simulink model "BEML_EMU"  (R2019b)
settings: configuration reference "ConfigSet_SimIntegration" (kept outside this file)
model workspace (MAT data in the model file):
  BrakesSampleTime = 0.01
  ConfigSampleTime = 0.05
  CouplingSampleTime = 0.05
  DoorsSampleTime = 0.05
  DynamicsSampleTime = 0.001
  ElectricalSampleTime = 0.05
  PRM_SimIntegration : Simulink.Parameter (value not decoded)
  PantographSampleTime = 0.05
  PneumaticsSampleTime = 0.01
  SampleTime = 0.001
  TractionSampleTime = 0.01
undefined symbols (not defined in the file): Acceleration, AngularAcceleration, AngularVelocity, BrakeFadeEnable, Brakes, BrakeShoeCoefficientCalculationMethod, BrakeShoeFrictionCoeff, BrakeTemperatureEnable, Common, DampingAdjustmentDesignMass, DavisCoeffA1, DavisCoeffA2, DavisCoeffB1, DavisCoeffB2, DavisCoefficients, DavisCoeffLeadCarC, DavisCoeffTailCarC, DiscIntNeverNeededParam, Doors, DragCalculationMethod, Dynamics, Effects, Electrical, EnableDampingAdjustmentByMass, Environment, Equipment, ExternalEffects, H, HasMotor, HasPanto, HornActivation, IsFirstVehicle, IsLastVehicle, isLeft, IsNonCab, LateralJolt, Location, LongitudinalJolt, MaxVehicles, MotionBaseSafetyCutout, OrientationDCM, P, Pantograph, Pneumatics, PneumaticsPoweredPanto, R, Traction, Transform, Tuning, UnitConfig, Velocity, VerticalJolt, VerticalJoltDown, VigilanceIntervention
libraries: simulink x35, IOStateMachinesLib x26, TestBenchLib x6, LatchesLib x3, BEML_EMU_BrakesInput_Lib x1, BEML_EMU_CBTCInterface_Lib x1, BEML_EMU_Couplers_Lib x1, BEML_EMU_DoorsInput_Lib x1, BEML_EMU_DynamicsInput_Lib x1, BEML_EMU_ElectricalInput_Lib x1, BEML_EMU_PantographInput_Lib x1, BEML_EMU_PneumaticsInput_Lib x1
(part 3 of 6)

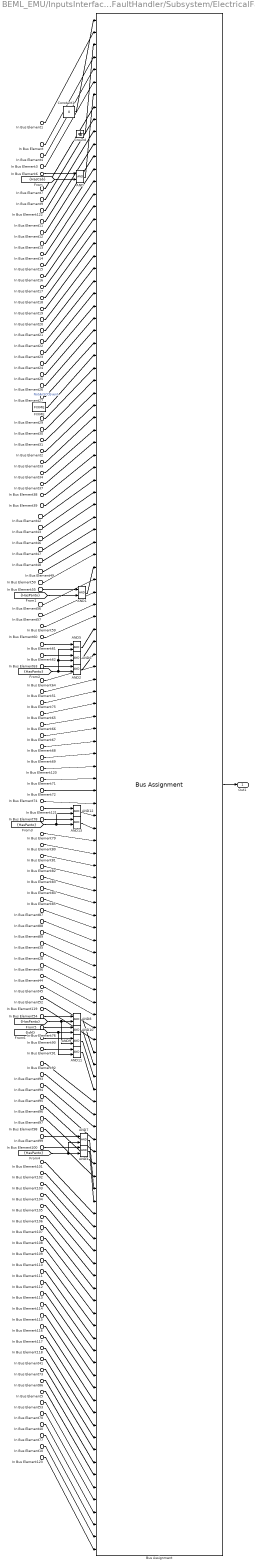
== system BEML_EMU/InputsInterface/FaultHandler/Subsystem/ElectricalFaults ==
  In Bus Element4 : Inport  PortName=TrainFaults  Element=FWDREVTrainLineMismatch
  In Bus Element6 : Inport  PortName=TrainFaults  Element=LowMRPressure
  In Bus Element7 : Inport  PortName=TrainFaults  Element=ReverseMotionInForwardCommand
  In Bus Element9 : Inport  PortName=TrainFaults  Element=InternalFireAlarmTLActive
  In Bus Element11 : Inport  PortName=TrainFaults  Element=TractionCutModeSelectorInATPATOUTO
  In Bus Element12 : Inport  PortName=TrainFaults  Element=DamagedOHE
  In Bus Element13 : Inport  PortName=TrainFaults  Element=DoorsNotOpeningFromDOPBOP1
  In Bus Element14 : Inport  PortName=TrainFaults  Element=DepotSignalMalfunction
  In Bus Element15 : Inport  PortName=TrainFaults  Element=TrackCircuitOccupied
  In Bus Element16 : Inport  PortName=TrainFaults  Element=MainSignalSwitchesToRed
  In Bus Element17 : Inport  PortName=TrainFaults  Element=PlatformScreenDoorNotWorking
  In Bus Element18 : Inport  PortName=TrainFaults  Element=TrainGettingZeroSpeedOrder
  In Bus Element19 : Inport  PortName=TrainFaults  Element=ATCEBUnableToReset
  In Bus Element20 : Inport  PortName=TrainFaults  Element=TrainOvershootATCNotAllowingReverseAlignment
  In Bus Element21 : Inport  PortName=TrainFaults  Element=FSBAppliedAt10KMPH
  In Bus Element122 : Inport  PortName=TrainFaults  Element=FDUFaultAlarmTLActive
  In Bus Element1 : Inport  Port=2  PortName=VehicleFaults  Element=PantographDownForADDIntervention
  In Bus Element : Inport  Port=2  PortName=VehicleFaults  Element=PantographRaiseFailure
  In Bus Element3 : Inport  Port=2  PortName=VehicleFaults  Element=CCDetectDetrainmentDoorOpen
  In Bus Element22 : Inport  Port=2  PortName=VehicleFaults  Element=HVAC1SupplyFanMPCBTrip
  In Bus Element23 : Inport  Port=2  PortName=VehicleFaults  Element=HVAC1EmergencyInverterTrip
  In Bus Element24 : Inport  Port=2  PortName=VehicleFaults  Element=HVAC1RCCBTrip
  In Bus Element25 : Inport  Port=2  PortName=VehicleFaults  Element=HVAC1FireMode
  In Bus Element26 : Inport  Port=2  PortName=VehicleFaults  Element=HVAC1ExternalSmokeMode
  In Bus Element27 : Inport  Port=2  PortName=VehicleFaults  Element=HVAC1ReducedMode
  In Bus Element29 : Inport  Port=2  PortName=VehicleFaults  Element=WFLFailure
  In Bus Element30 : Inport  Port=2  PortName=VehicleFaults  Element=ODDFailure
  In Bus Element31 : Inport  Port=2  PortName=VehicleFaults  Element=ObstacleDetectedRightSide
  In Bus Element33 : Inport  Port=2  PortName=VehicleFaults  Element=CouplingCircuitNotPowered
  In Bus Element34 : Inport  Port=2  PortName=VehicleFaults  Element=CabEnablingCircuitBreakerTripped
  In Bus Element37 : Inport  Port=2  PortName=VehicleFaults  Element=OHLHighVoltageLevel3
  In Bus Element38 : Inport  Port=2  PortName=VehicleFaults  Element=OHLLowVoltageLevel2
  In Bus Element39 : Inport  Port=2  PortName=VehicleFaults  Element=LineConverterOverCurrentLevel2
  In Bus Element42 : Inport  Port=2  PortName=VehicleFaults  Element=LineConverterIGBTFailure
  In Bus Element43 : Inport  Port=2  PortName=VehicleFaults  Element=DC110VLowVoltage
  In Bus Element46 : Inport  Port=2  PortName=VehicleFaults  Element=OverTemperatureOfInverterPowerUnit
  In Bus Element47 : Inport  Port=2  PortName=VehicleFaults  Element=OverTemperatureOfConverterPowerUnit
  In Bus Element48 : Inport  Port=2  PortName=VehicleFaults  Element=AKOpenFailure
  In Bus Element49 : Inport  Port=2  PortName=VehicleFaults  Element=KOpenFailure
  In Bus Element50 : Inport  Port=2  PortName=VehicleFaults  Element=MainCircuitEarthFaultLevel2
  In Bus Element55 : Inport  Port=2  PortName=VehicleFaults  Element=VCBOpenedByCI
  In Bus Element56 : Inport  Port=2  PortName=VehicleFaults  Element=PantographDownForBUVDRIntervention
  In Bus Element57 : Inport  Port=2  PortName=VehicleFaults  Element=PantographCircuitNotEnergized
  In Bus Element59 : Inport  Port=2  PortName=VehicleFaults  Element=TransformerOilPressureTooLow
  In Bus Element60 : Inport  Port=2  PortName=VehicleFaults  Element=TransformerOilTemperatureTooHigh
  In Bus Element61 : Inport  Port=2  PortName=VehicleFaults  Element=VCBOpenedByACOvercurrent
  In Bus Element62 : Inport  Port=2  PortName=VehicleFaults  Element=VCBOpenedByMTrProtection
  In Bus Element63 : Inport  Port=2  PortName=VehicleFaults  Element=VCBOpenedByAPS
  In Bus Element64 : Inport  Port=2  PortName=VehicleFaults  Element=PantographLoweringFailure
  In Bus Element65 : Inport  Port=2  PortName=VehicleFaults  Element=MCB110VDCGroupTripped
  In Bus Element66 : Inport  Port=2  PortName=VehicleFaults  Element=MechanicalCouplerRelayFault
  In Bus Element67 : Inport  Port=2  PortName=VehicleFaults  Element=BatteryFuseBlown
  In Bus Element68 : Inport  Port=2  PortName=VehicleFaults  Element=BICContactorActivationFault
  In Bus Element69 : Inport  Port=2  PortName=VehicleFaults  Element=LowBatteryVoltageAlarm
  In Bus Element71 : Inport  Port=2  PortName=VehicleFaults  Element=MCBHVACGroupTripped
  In Bus Element72 : Inport  Port=2  PortName=VehicleFaults  Element=HVAC1MajorFault
  In Bus Element74 : Inport  Port=2  PortName=VehicleFaults  Element=MCBSignalingGroupTripped
  In Bus Element78 : Inport  Port=2  PortName=VehicleFaults  Element=APSCircuitBreakerTripped
  In Bus Element79 : Inport  Port=2  PortName=VehicleFaults  Element=SmokeAlarmCABArea
  In Bus Element80 : Inport  Port=2  PortName=VehicleFaults  Element=HeatAlarmEDB
  In Bus Element81 : Inport  Port=2  PortName=VehicleFaults  Element=TrainRadioFailure
  In Bus Element82 : Inport  Port=2  PortName=VehicleFaults  Element=PEA1AlarmActive
  In Bus Element83 : Inport  Port=2  PortName=VehicleFaults  Element=PEA1CallNotAcknowledged
  In Bus Element84 : Inport  Port=2  PortName=VehicleFaults  Element=PEA1Failure
  In Bus Element85 : Inport  Port=2  PortName=VehicleFaults  Element=MCBPAGroupOpen
  In Bus Element87 : Inport  Port=2  PortName=VehicleFaults  Element=CommunicationErrorRIO1RIO2
  In Bus Element88 : Inport  Port=2  PortName=VehicleFaults  Element=MCBTCMSGroupTripped
  In Bus Element89 : Inport  Port=2  PortName=VehicleFaults  Element=ER1MajorFault
  In Bus Element51 : Inport  Port=2  PortName=VehicleFaults  Element=MCBBrakeGroupTripped
  In Bus Element75 : Inport  Port=2  PortName=VehicleFaults  Element=MCBDoorGroupTripped
  In Bus Element35 : Inport  Port=2  PortName=VehicleFaults  Element=EDNORDeactivatedInRunningTrain
  In Bus Element28 : Inport  Port=2  PortName=VehicleFaults  Element=AllDoorCloseIndicatorNotWorking
  In Bus Element36 : Inport  Port=2  PortName=VehicleFaults  Element=TrainDoorLockedClosedRelayFailure
  In Bus Element44 : Inport  Port=2  PortName=VehicleFaults  Element=WipersNotWorking
  In Bus Element45 : Inport  Port=2  PortName=VehicleFaults  Element=FloodLightNotWorking
  In Bus Element52 : Inport  Port=2  PortName=VehicleFaults  Element=ShutdownFailureVCBOpening
  In Bus Element54 : Inport  Port=2  PortName=VehicleFaults  Element=ExteriorLight1CBTripped
  In Bus Element76 : Inport  Port=2  PortName=VehicleFaults  Element=ExteriorLight2CBTripped
  In Bus Element90 : Inport  Port=2  PortName=VehicleFaults  Element=InteriorLight1CBTripped
  In Bus Element91 : Inport  Port=2  PortName=VehicleFaults  Element=InteriorLight2CBTripped
  In Bus Element92 : Inport  Port=2  PortName=VehicleFaults  Element=CMCContactorActivationFailure
  In Bus Element93 : Inport  Port=2  PortName=VehicleFaults  Element=CMCContactorDeactivationFailure
  In Bus Element94 : Inport  Port=2  PortName=VehicleFaults  Element=APSGroup1Failure
  In Bus Element95 : Inport  Port=2  PortName=VehicleFaults  Element=APSGroup1Isolated
  In Bus Element96 : Inport  Port=2  PortName=VehicleFaults  Element=BCGGroup1Failure
  In Bus Element97 : Inport  Port=2  PortName=VehicleFaults  Element=BCGGroup1IsolationFailure
  In Bus Element98 : Inport  Port=2  PortName=VehicleFaults  Element=BCGGroup1Isolated
  In Bus Element99 : Inport  Port=2  PortName=VehicleFaults  Element=VCBMissingClosing
  In Bus Element100 : Inport  Port=2  PortName=VehicleFaults  Element=VCBMissingOpening
  In Bus Element101 : Inport  Port=2  PortName=VehicleFaults  Element=HeadlightFailure
  In Bus Element102 : Inport  Port=2  PortName=VehicleFaults  Element=HornBlowsContinuously
  In Bus Element103 : Inport  Port=2  PortName=VehicleFaults  Element=LineVoltageIndicatorNotWorking
  In Bus Element104 : Inport  Port=2  PortName=VehicleFaults  Element=OtherCabOccupiedIndicatorFaulty
  In Bus Element105 : Inport  Port=2  PortName=VehicleFaults  Element=DoorClosePBOP1NotWorking
  In Bus Element106 : Inport  Port=2  PortName=VehicleFaults  Element=EmergencyBrakePBOP1NotWorking
  In Bus Element107 : Inport  Port=2  PortName=VehicleFaults  Element=DoorCloseAnnouncementPBNotWorking
  In Bus Element108 : Inport  Port=2  PortName=VehicleFaults  Element=FailureOfTrainborneATCEquipment
  In Bus Element109 : Inport  Port=2  PortName=VehicleFaults  Element=DMIFailure
  In Bus Element110 : Inport  Port=2  PortName=VehicleFaults  Element=TransformerOilLevelLow
  In Bus Element111 : Inport  Port=2  PortName=VehicleFaults  Element=TransformerOilFlowWarning
  In Bus Element112 : Inport  Port=2  PortName=VehicleFaults  Element=TransformerOilPressureWarning
  In Bus Element113 : Inport  Port=2  PortName=VehicleFaults  Element=TransformerOilTemperatureHigh
  In Bus Element114 : Inport  Port=2  PortName=VehicleFaults  Element=PCUFailure
  In Bus Element115 : Inport  Port=2  PortName=VehicleFaults  Element=PEA2Failure
  In Bus Element116 : Inport  Port=2  PortName=VehicleFaults  Element=PEA3Failure
  In Bus Element117 : Inport  Port=2  PortName=VehicleFaults  Element=SCU2Failure
  In Bus Element118 : Inport  Port=2  PortName=VehicleFaults  Element=EBNotReleased
  In Bus Element41 : Inport  Port=2  PortName=VehicleFaults  Element=CIMicroprocessorAbnormal
  In Bus Element73 : Inport  Port=2  PortName=VehicleFaults  Element=CILocalCommunicationFailure
  In Bus Element86 : Inport  Port=2  PortName=VehicleFaults  Element=TransformerOilLevelTooLow
  In Bus Element119 : Inport  Port=2  PortName=VehicleFaults  Element=MCBLightGroupSaloonTripped
  In Bus Element120 : Inport  Port=2  PortName=VehicleFaults  Element=MCBLightGroupTripped
  In Bus Element121 : Inport  Port=2  PortName=VehicleFaults  Element=MCBAPSGroupTripped
  In Bus Element5 : Inport  Port=2  PortName=VehicleFaults  Element=PantographRisingMissing
  In Bus Element53 : Inport  Port=2  PortName=VehicleFaults  Element=PantographLoweringMissing
  In Bus Element70 : Inport  Port=2  PortName=VehicleFaults  Element=PantographRisingInhibited
  In Bus Element40 : Inport  Port=2  PortName=VehicleFaults  Element=CIFailure
  In Bus Element77 : Inport  Port=2  PortName=VehicleFaults  Element=CIIsolated
  In Bus Element10 : Inport  Port=2  PortName=VehicleFaults  Element=EmergencyBrakeDueToEBPB
  In Bus Element123 : Inport  Port=2  PortName=VehicleFaults  Element=EmergencyBrakeDueDeadman
  In Bus Element2 : Inport  Port=2  PortName=VehicleFaults  Element=DerailmentDetectedRightSide
  AND{,1..2,4..13} (13 alike) : Logic  AllPortsSameDT=off  OutDataTypeStr=boolean
  Bus Assignment : BusAssignment  AssignedSignals=PantographDownForADDIntervention,PantographDownForORDIntervention,PantographRisingFailure,FwdRevTrainLineMismatch,CCDetectedEmerDoorOpen,LowMRPressure,ReverseMotionInForwardCommand,InternalFireAlarmTLActive,FDUFailure,TractionCutModeSelectorInATPATOUTO,DamagedOHE,DoorsNotOpeningFromDOPBOP1,DepotSignalMalfunction,TrackCircuitOccupied,MainSignalSwitchesToRed,PlatformScreenDoorNotWorking,TrainGettingZeroSpeedOrder,ATCEBUnableToReset,TrainOvershootATCNotAllowingReverseAlignment,FSBAppliedAt10KMPH,HVAC1SupplyFanMPCBTrip,HVAC1EmergencyInverterTrip,HVAC1RCCBTrip,HVAC1FireMode,HVAC1ExternalSmokeMode,HVAC1ReducedMode,CabSaloonPartitionDoorOpen,WFLFailure,ODDFailure,ObstacleDetectedRightSide,DerailmentDetectedRightSide,CouplingCircuitNotPowered,CabEnablingCircuitBreakerTripped,OHLHighVoltageLevel3,OHLLowVoltageLevel2,LineConverterOverCurrentLevel2,LineConverterIGBTFailure,DC110VLowVoltage,OverTemperatureOfInverterPowerUnit,OverTemperatureOfConverterPowerUnit,AKOpenFailure,KOpenFailure,MainCircuitEarthFaultLevel2,VCBOpenedByCI,PantographDownForBUVDRIntervention,PantographCircuitNotEnergized,TransformerOilPressureTooLow,TransformerOilTemperatureTooHigh,VCBOpenedByACOvercurrent,VCBOpenedByMTrProtection,VCBOpenedByAPS,PantographLoweringFailure,MCBBrakeGroupTripped,MCBDoorGroupTripped,MCB110VDCGroupTripped,MechanicalCouplerRelayFault,BatteryFuseBlown,BICContactorActivationFault,LowBatteryVoltageAlarm,LightGroupMCBTripped,MCBHVACGroupTripped,HVAC1MajorFault,MCBSignalingGroupTripped,APSMCBGroupTripped,APSCircuitBreakerTripped,SmokeAlarmCABArea,HeatAlarmEDB,TrainRadioFailure,PEA1AlarmActive,PEA1CallNotAcknowledged,PEA1Failure,MCBPAGroupOpen,CommunicationErrorRIO1RIO2,MCBTCMSGroupTripped,ER1MajorFault,EmerDoorNotOpenRelayDeactivated,AllDoorCloseIndicatorNotWorking,TrainDoorLockedClosedRelayFailure,WipersNotWorking,FloodLightNotWorking,ShutdownFailureVCBOpening,LightGroupSaloonMCBTripped,ExteriorLight1CBTripped,ExteriorLight2CBTripped,InteriorLight1CBTripped,InteriorLight2CBTripped,CMCContactorActivationFailure,CMCContactorDeactivationFailure,APSGroup1Failure,APSGroup1Isolated,BCGGroup1Failure,BCGGroup1IsolationFailure,BCGGroup1Isolated,VCBMissingClosing,VCBMissingOpening,HeadlightFailure,HornBlowsContinuously,LineVoltageIndicatorNotWorking,OtherCabOccupiedIndicatorFaulty,DoorClosePBOP1NotWorking,EmergencyBrakePBOP1NotWorking,DoorCloseAnnouncementPBNotWorking,ATCFailure,DMIFailure,TransformerOilLevelLow,TransformerOilFlowWarning,TransformerOilPressureWarning,TransformerOilTemperatureHigh,PCUFailure,PEA2Failure,PEA3Failure,SCU2Failure,EBNotReleased,CIMicroprocessorAbnormal,CILocalCommunicationFailure,TransformerOilLevelTooLow,PantographRisingMissing,PantographLoweringMissing,PantographRisingInhibited,CIFailure,CIIsolated,EmergencyBrakeDueToEBPB,EmergencyBrakeDueDeadman
  Constant1 : Constant  Value=0  OutDataTypeStr=Bus: BD_ElectricalSystem_In_Faults
  FIXME : TestBenchLib/FIXME
      settings: SourceProductName=Sydac Utilities
  Ground : Ground
  Out1 : Outport
  wires:
  Bus Assignment/1 -> Out1/1
  Constant1/1 -> Bus Assignment/1
  In Bus Element1/1 -> Bus Assignment/2
  In Bus Element/1 -> Bus Assignment/4
  In Bus Element3/1 -> Bus Assignment/6
  In Bus Element6/1 -> AND/1
  AND/1 -> Bus Assignment/7
  [HasCab] -> AND/2
  In Bus Element55/1 -> AND1/1
  [HasPanto] -> AND1/2
  In Bus Element7/1 -> Bus Assignment/8
  In Bus Element61/1 -> AND5/1
  In Bus Element78/1 -> AND13/1
  In Bus Element99/1 -> AND7/1
  In Bus Element62/1 -> AND6/1
  [HasPanto] -> AND9/2, AND8/2
  In Bus Element54/1 -> AND8/1
  [HasPanto] -> AND12/2, AND13/2
  [HasPanto] -> AND6/2, AND5/2, AND2/2
  [HasPanto] -> AND7/2, AND4/2
  [IsM] -> AND11/2, AND10/2
  In Bus Element91/1 -> AND11/1
  In Bus Element121/1 -> AND12/1
  In Bus Element76/1 -> AND10/1
  In Bus Element90/1 -> AND9/1
  In Bus Element63/1 -> AND2/1
  In Bus Element100/1 -> AND4/1
  In Bus Element2/1 -> Bus Assignment/32
  FIXME/1 -> Bus Assignment/28  "NotAnSCCEvent"
  In Bus Element9/1 -> Bus Assignment/9
  In Bus Element122/1 -> Bus Assignment/10
  In Bus Element11/1 -> Bus Assignment/11
  In Bus Element12/1 -> Bus Assignment/12
  In Bus Element13/1 -> Bus Assignment/13
  In Bus Element14/1 -> Bus Assignment/14
  In Bus Element15/1 -> Bus Assignment/15
  In Bus Element16/1 -> Bus Assignment/16
  In Bus Element17/1 -> Bus Assignment/17
  In Bus Element18/1 -> Bus Assignment/18
  In Bus Element19/1 -> Bus Assignment/19
  In Bus Element20/1 -> Bus Assignment/20
  In Bus Element21/1 -> Bus Assignment/21
  In Bus Element22/1 -> Bus Assignment/22
  In Bus Element23/1 -> Bus Assignment/23
  In Bus Element24/1 -> Bus Assignment/24
  In Bus Element25/1 -> Bus Assignment/25
  In Bus Element26/1 -> Bus Assignment/26
  In Bus Element27/1 -> Bus Assignment/27
  In Bus Element29/1 -> Bus Assignment/29
  In Bus Element30/1 -> Bus Assignment/30
  In Bus Element33/1 -> Bus Assignment/33
  In Bus Element34/1 -> Bus Assignment/34
  In Bus Element37/1 -> Bus Assignment/35
  In Bus Element38/1 -> Bus Assignment/36
  In Bus Element39/1 -> Bus Assignment/37
  In Bus Element42/1 -> Bus Assignment/38
  In Bus Element43/1 -> Bus Assignment/39
  In Bus Element46/1 -> Bus Assignment/40
  In Bus Element47/1 -> Bus Assignment/41
  In Bus Element48/1 -> Bus Assignment/42
  In Bus Element49/1 -> Bus Assignment/43
  In Bus Element50/1 -> Bus Assignment/44
  AND1/1 -> Bus Assignment/45
  AND5/1 -> Bus Assignment/50
  AND6/1 -> Bus Assignment/51
  AND2/1 -> Bus Assignment/52
  In Bus Element59/1 -> Bus Assignment/48
  In Bus Element60/1 -> Bus Assignment/49
  In Bus Element56/1 -> Bus Assignment/46
  In Bus Element57/1 -> Bus Assignment/47
  In Bus Element64/1 -> Bus Assignment/53
  In Bus Element51/1 -> Bus Assignment/54
  In Bus Element75/1 -> Bus Assignment/55
  In Bus Element65/1 -> Bus Assignment/56
  In Bus Element66/1 -> Bus Assignment/57
  In Bus Element67/1 -> Bus Assignment/58
  In Bus Element68/1 -> Bus Assignment/59
  In Bus Element69/1 -> Bus Assignment/60
  In Bus Element120/1 -> Bus Assignment/61
  In Bus Element71/1 -> Bus Assignment/62
  In Bus Element72/1 -> Bus Assignment/63
  In Bus Element74/1 -> Bus Assignment/64
  AND12/1 -> Bus Assignment/65
  AND13/1 -> Bus Assignment/66
  AND8/1 -> Bus Assignment/84
  AND10/1 -> Bus Assignment/85
  AND9/1 -> Bus Assignment/86
  AND11/1 -> Bus Assignment/87
  In Bus Element79/1 -> Bus Assignment/67
  In Bus Element80/1 -> Bus Assignment/68
  In Bus Element81/1 -> Bus Assignment/69
  In Bus Element82/1 -> Bus Assignment/70
  In Bus Element83/1 -> Bus Assignment/71
  In Bus Element84/1 -> Bus Assignment/72
  In Bus Element85/1 -> Bus Assignment/73
  In Bus Element87/1 -> Bus Assignment/74
  In Bus Element88/1 -> Bus Assignment/75
  In Bus Element89/1 -> Bus Assignment/76
  In Bus Element35/1 -> Bus Assignment/77
  In Bus Element28/1 -> Bus Assignment/78
  In Bus Element36/1 -> Bus Assignment/79
  In Bus Element44/1 -> Bus Assignment/80
  In Bus Element45/1 -> Bus Assignment/81
  In Bus Element52/1 -> Bus Assignment/82
  In Bus Element119/1 -> Bus Assignment/83
  AND7/1 -> Bus Assignment/95
  AND4/1 -> Bus Assignment/96
  In Bus Element92/1 -> Bus Assignment/88
  In Bus Element93/1 -> Bus Assignment/89
  In Bus Element94/1 -> Bus Assignment/90
  In Bus Element95/1 -> Bus Assignment/91
  In Bus Element96/1 -> Bus Assignment/92
  In Bus Element97/1 -> Bus Assignment/93
  In Bus Element98/1 -> Bus Assignment/94
  In Bus Element101/1 -> Bus Assignment/97
  In Bus Element102/1 -> Bus Assignment/98
  In Bus Element103/1 -> Bus Assignment/99
  In Bus Element104/1 -> Bus Assignment/100
  In Bus Element105/1 -> Bus Assignment/101
  In Bus Element106/1 -> Bus Assignment/102
  In Bus Element107/1 -> Bus Assignment/103
  In Bus Element108/1 -> Bus Assignment/104
  In Bus Element109/1 -> Bus Assignment/105
  In Bus Element110/1 -> Bus Assignment/106
  In Bus Element111/1 -> Bus Assignment/107
  In Bus Element112/1 -> Bus Assignment/108
  In Bus Element113/1 -> Bus Assignment/109
  In Bus Element114/1 -> Bus Assignment/110
  In Bus Element115/1 -> Bus Assignment/111
  In Bus Element116/1 -> Bus Assignment/112
  In Bus Element117/1 -> Bus Assignment/113
  In Bus Element118/1 -> Bus Assignment/114
  In Bus Element41/1 -> Bus Assignment/115
  In Bus Element73/1 -> Bus Assignment/116
  In Bus Element86/1 -> Bus Assignment/117
  In Bus Element5/1 -> Bus Assignment/118
  In Bus Element53/1 -> Bus Assignment/119
  In Bus Element70/1 -> Bus Assignment/120
  In Bus Element40/1 -> Bus Assignment/121
  In Bus Element77/1 -> Bus Assignment/122
  In Bus Element10/1 -> Bus Assignment/123
  In Bus Element123/1 -> Bus Assignment/124
  In Bus Element4/1 -> Bus Assignment/5
  Ground/1 -> Bus Assignment/3
  In Bus Element31/1 -> Bus Assignment/31

== system BEML_EMU/InputsInterface/FaultHandler/Subsystem/PantographFaults ==
  In Bus Element : Inport  PortName=VehicleFaults  Element=PantographDownForADDIntervention
  Bus Assignment : BusAssignment  AssignedSignals=PlaceHolder
  Constant1 : Constant  Value=0  OutDataTypeStr=Bus: BD_PantographSystem_In_Vehicle_Faults
  Out1 : Outport
  wires:
  Bus Assignment/1 -> Out1/1
  Constant1/1 -> Bus Assignment/1
  In Bus Element/1 -> Bus Assignment/2

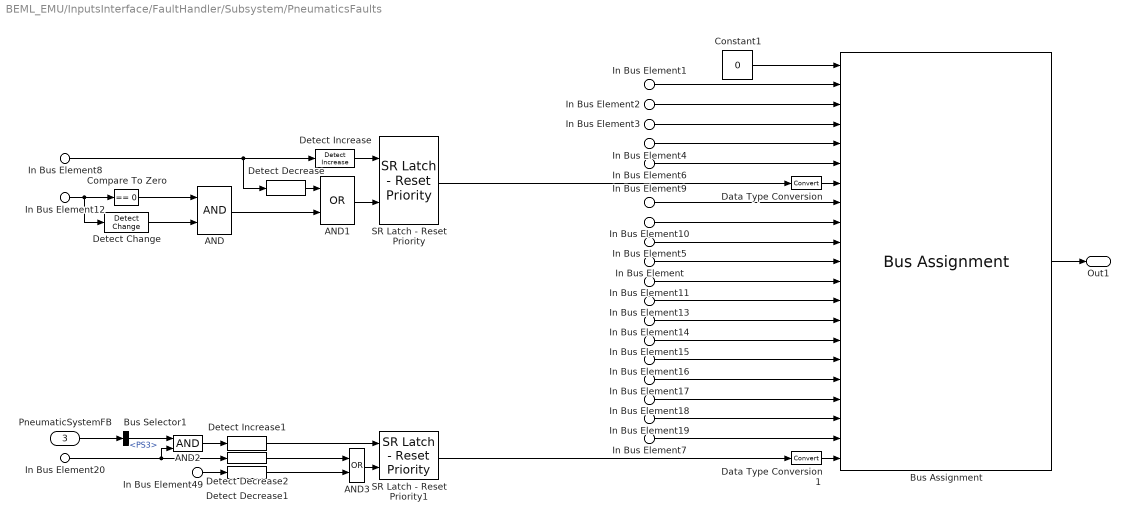
== system BEML_EMU/InputsInterface/FaultHandler/Subsystem/PneumaticsFaults ==
  In Bus Element1 : Inport  PortName=VehicleFaults  Element=HeavyWheelSlip
  In Bus Element2 : Inport  PortName=VehicleFaults  Element=BECU1AxleLockedWheelSet1
  In Bus Element3 : Inport  PortName=VehicleFaults  Element=BECU1ServiceBrakeFailure
  In Bus Element4 : Inport  PortName=VehicleFaults  Element=BECU1EmergencyBrakeFailure
  In Bus Element5 : Inport  PortName=VehicleFaults  Element=BECUMajorFault
  In Bus Element6 : Inport  PortName=VehicleFaults  Element=AirSuspensionBogie1Deflated
  In Bus Element8 : Inport  PortName=VehicleFaults  Element=BrakeDemandSignalFailure
  In Bus Element9 : Inport  PortName=VehicleFaults  Element=ParkingBrakeApplicationFailure
  In Bus Element10 : Inport  PortName=VehicleFaults  Element=ParkingBrakeReleaseFailure
  In Bus Element : Inport  PortName=VehicleFaults  Element=PressureGuageNotWorking
  In Bus Element11 : Inport  PortName=VehicleFaults  Element=PantographPipeLowPressure
  In Bus Element13 : Inport  PortName=VehicleFaults  Element=BECU2AxleLockedWheelSet2
  In Bus Element14 : Inport  PortName=VehicleFaults  Element=BECU2EmergencyBrakeFailure
  In Bus Element15 : Inport  PortName=VehicleFaults  Element=BECU1BrakeNotApplied
  In Bus Element16 : Inport  PortName=VehicleFaults  Element=BECU1BrakeNotReleased
  In Bus Element17 : Inport  PortName=VehicleFaults  Element=BECU1CarLoadPressureLow
  In Bus Element18 : Inport  PortName=VehicleFaults  Element=BECU2CarLoadPressureLow
  In Bus Element19 : Inport  PortName=VehicleFaults  Element=BECULowRPressure
  In Bus Element7 : Inport  PortName=VehicleFaults  Element=BECU1LoadPressureLow
  In Bus Element20 : Inport  PortName=VehicleFaults  Element=PantographDownForORDIntervention
  In Bus Element12 : Inport  Port=2  PortName=InputControlStates  Element=ModeSelector
  In Bus Element49 : Inport  Port=2  PortName=InputControlStates  Element=ORDPlunger
  PneumaticSystemFB : Inport  Port=3
  AND : Logic  AllPortsSameDT=off  OutDataTypeStr=boolean
  AND1 : Logic  Operator=OR  AllPortsSameDT=off  OutDataTypeStr=boolean
  AND2 : Logic  AllPortsSameDT=off  OutDataTypeStr=boolean
  AND3 : Logic  Operator=OR  AllPortsSameDT=off  OutDataTypeStr=boolean
  Bus Assignment : BusAssignment  AssignedSignals=HeavyWheelSlip,BECU1AxleLockedWheelSet1,BECU1ServiceBrakeFailure,BECU1EmergencyBrakeFailure,AirSuspensionBogie1Deflated,BrakeDemandSignalFailure,ParkingBrakeApplicationFailure,ParkingBrakeReleaseFailure,BECUMajorFault,PressureGuageNotWorking,PantographPipeLowPressure,BECU2AxleLockedWheelSet2,BECU2EmergencyBrakeFailure,BECU1BrakeNotApplied,BECU1BrakeNotReleased,BECU1CarLoadPressureLow,BECU2CarLoadPressureLow,BECULowRPressure,BECU1LoadPressureLow,ORDIntervention
  Bus Selector1 : BusSelector  OutputSignals=PressureSwitches.PS3
  Compare To Zero : simulink/Logic and Bit Operations/Compare To Zero  relop===  OutDataTypeStr=boolean
  Constant1 : Constant  Value=0  OutDataTypeStr=Bus: BD_PneumaticsSystem_In_Vehicle_Faults
  Data Type Conversion : DataTypeConversion
  Data Type Conversion1 : DataTypeConversion
  Detect Change : simulink/Logic and Bit Operations/Detect Change  vinit=0  OutDataTypeStr=boolean
  Detect Decrease : simulink/Logic and Bit Operations/Detect Decrease  vinit=0.0  OutDataTypeStr=boolean
  Detect Decrease1 : simulink/Logic and Bit Operations/Detect Decrease  vinit=0.0  OutDataTypeStr=boolean
  Detect Decrease2 : simulink/Logic and Bit Operations/Detect Decrease  vinit=0.0  OutDataTypeStr=boolean
  Detect Increase : simulink/Logic and Bit Operations/Detect Increase  vinit=0.0  OutDataTypeStr=boolean
  Detect Increase1 : simulink/Logic and Bit Operations/Detect Increase  vinit=0.0  OutDataTypeStr=boolean
  SR Latch - Reset Priority : LatchesLib/SR Latch - Reset Priority  initial_condition=0
      settings: SourceProductName=Latches
  SR Latch - Reset Priority1 : LatchesLib/SR Latch - Reset Priority  initial_condition=0
      settings: SourceProductName=Latches
  Out1 : Outport
  wires:
  Constant1/1 -> Bus Assignment/1
  Bus Assignment/1 -> Out1/1
  In Bus Element1/1 -> Bus Assignment/2
  In Bus Element2/1 -> Bus Assignment/3
  In Bus Element3/1 -> Bus Assignment/4
  In Bus Element4/1 -> Bus Assignment/5
  In Bus Element6/1 -> Bus Assignment/6
  SR Latch - Reset Priority/1 -> Data Type Conversion/1
  In Bus Element8/1 -> Detect Decrease/1, Detect Increase/1
  In Bus Element12/1 -> Detect Change/1, Compare To Zero/1
  Detect Increase/1 -> SR Latch - Reset Priority/1
  Compare To Zero/1 -> AND/1
  AND/1 -> AND1/2
  Detect Change/1 -> AND/2
  AND1/1 -> SR Latch - Reset Priority/2
  Detect Decrease/1 -> AND1/1
  Data Type Conversion/1 -> Bus Assignment/7
  In Bus Element9/1 -> Bus Assignment/8
  In Bus Element10/1 -> Bus Assignment/9
  In Bus Element5/1 -> Bus Assignment/10
  In Bus Element/1 -> Bus Assignment/11
  In Bus Element11/1 -> Bus Assignment/12
  In Bus Element13/1 -> Bus Assignment/13
  In Bus Element14/1 -> Bus Assignment/14
  In Bus Element15/1 -> Bus Assignment/15
  In Bus Element16/1 -> Bus Assignment/16
  In Bus Element17/1 -> Bus Assignment/17
  In Bus Element18/1 -> Bus Assignment/18
  In Bus Element19/1 -> Bus Assignment/19
  In Bus Element7/1 -> Bus Assignment/20
  SR Latch - Reset Priority1/1 -> Data Type Conversion1/1
  In Bus Element49/1 -> Detect Decrease1/1
  Data Type Conversion1/1 -> Bus Assignment/21
  Detect Increase1/1 -> SR Latch - Reset Priority1/1
  Detect Decrease1/1 -> AND3/2
  Bus Selector1/1 -> AND2/1  "<PS3>"
  PneumaticSystemFB/1 -> Bus Selector1/1
  AND2/1 -> Detect Increase1/1
  Detect Decrease2/1 -> AND3/1
  AND3/1 -> SR Latch - Reset Priority1/2
  In Bus Element20/1 -> Detect Decrease2/1, AND2/2

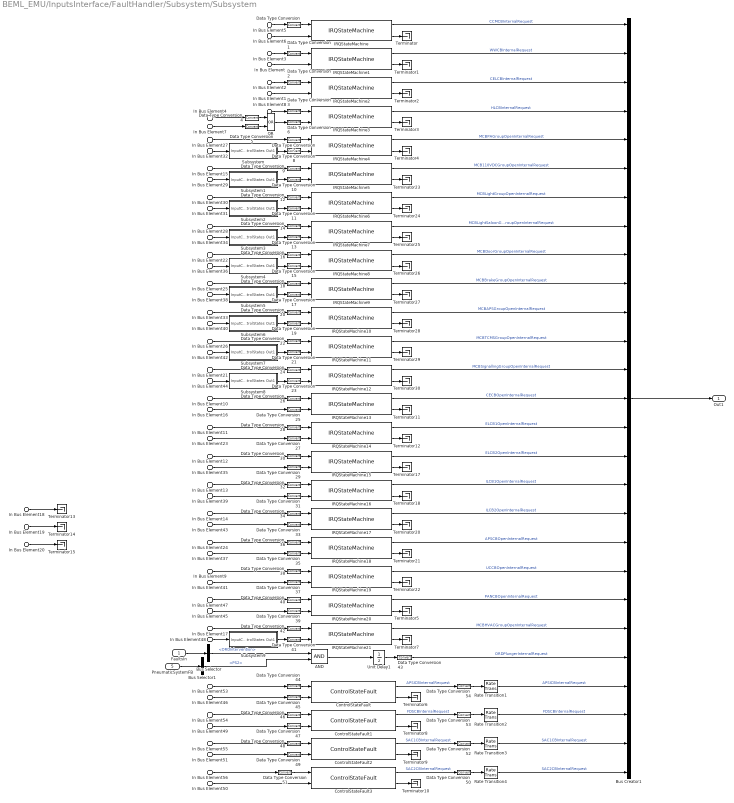
== system BEML_EMU/InputsInterface/FaultHandler/Subsystem/Subsystem ==
  FaultsIn : Inport
  In Bus Element5 : Inport  Port=2  PortName=TrainFaults  Element=LowMRPressure
  In Bus Element2 : Inport  Port=3  PortName=VehicleFaults  Element=FloodLightNotWorking
  In Bus Element3 : Inport  Port=3  PortName=VehicleFaults  Element=WipersNotWorking
  In Bus Element8 : Inport  Port=3  PortName=VehicleFaults  Element=HeadlightFailure
  In Bus Element10 : Inport  Port=3  PortName=VehicleFaults  Element=CabEnablingCircuitBreakerTripped
  In Bus Element11 : Inport  Port=3  PortName=VehicleFaults  Element=ExteriorLight1CBTripped
  In Bus Element12 : Inport  Port=3  PortName=VehicleFaults  Element=ExteriorLight2CBTripped
  In Bus Element13 : Inport  Port=3  PortName=VehicleFaults  Element=InteriorLight1CBTripped
  In Bus Element14 : Inport  Port=3  PortName=VehicleFaults  Element=InteriorLight2CBTripped
  In Bus Element15 : Inport  Port=3  PortName=VehicleFaults  Element=MCB110VDCGroupTripped
  In Bus Element17 : Inport  Port=3  PortName=VehicleFaults  Element=MCBHVACGroupTripped
  In Bus Element18 : Inport  Port=3  PortName=VehicleFaults  Element=HVAC1SupplyFanMPCBTrip
  In Bus Element19 : Inport  Port=3  PortName=VehicleFaults  Element=HVAC1EmergencyInverterTrip
  In Bus Element20 : Inport  Port=3  PortName=VehicleFaults  Element=HVAC1RCCBTrip
  In Bus Element21 : Inport  Port=3  PortName=VehicleFaults  Element=MCBSignalingGroupTripped
  In Bus Element22 : Inport  Port=3  PortName=VehicleFaults  Element=MCBDoorGroupTripped
  In Bus Element24 : Inport  Port=3  PortName=VehicleFaults  Element=APSCircuitBreakerTripped
  In Bus Element25 : Inport  Port=3  PortName=VehicleFaults  Element=MCBBrakeGroupTripped
  In Bus Element26 : Inport  Port=3  PortName=VehicleFaults  Element=MCBTCMSGroupTripped
  In Bus Element27 : Inport  Port=3  PortName=VehicleFaults  Element=MCBPAGroupOpen
  In Bus Element28 : Inport  Port=3  PortName=VehicleFaults  Element=MCBLightGroupSaloonTripped
  In Bus Element30 : Inport  Port=3  PortName=VehicleFaults  Element=MCBLightGroupTripped
  In Bus Element33 : Inport  Port=3  PortName=VehicleFaults  Element=MCBAPSGroupTripped
  In Bus Element9 : Inport  Port=3  PortName=VehicleFaults  Element=CouplingCircuitNotPowered
  In Bus Element47 : Inport  Port=3  PortName=VehicleFaults  Element=PantographCircuitNotEnergized
  In Bus Element{29,31..32,34,36,38,40,42,44,48} (10 alike) : Inport  Port=4  PortName=InputControlStates
  In Bus Element6 : Inport  Port=4  PortName=InputControlStates  Element=CMCCB
  In Bus Element : Inport  Port=4  PortName=InputControlStates  Element=WWCB
  In Bus Element1 : Inport  Port=4  PortName=InputControlStates  Element=CELCB
  In Bus Element4 : Inport  Port=4  PortName=InputControlStates  Element=HLLCB
  In Bus Element7 : Inport  Port=4  PortName=InputControlStates  Element=HLRCB
  In Bus Element16 : Inport  Port=4  PortName=InputControlStates  Element=CECB
  In Bus Element23 : Inport  Port=4  PortName=InputControlStates  Element=ELCB1
  In Bus Element35 : Inport  Port=4  PortName=InputControlStates  Element=ELCB2
  In Bus Element39 : Inport  Port=4  PortName=InputControlStates  Element=ILCB1
  In Bus Element43 : Inport  Port=4  PortName=InputControlStates  Element=ILCB2
  In Bus Element37 : Inport  Port=4  PortName=InputControlStates  Element=APSCB
  In Bus Element41 : Inport  Port=4  PortName=InputControlStates  Element=VCCBOrUCCB
  In Bus Element45 : Inport  Port=4  PortName=InputControlStates  Element=PANCB
  In Bus Element46 : Inport  Port=4  PortName=InputControlStates  Element=APSICB
  In Bus Element49 : Inport  Port=4  PortName=InputControlStates  Element=FDSCB
  In Bus Element50 : Inport  Port=4  PortName=InputControlStates  Element=SAC2CCB
  In Bus Element51 : Inport  Port=4  PortName=InputControlStates  Element=SAC1CCB
  PneumaticSystemFB : Inport  Port=5
  In Bus Element53 : Inport  Port=6  PortName=TCMSSystemFB  Element=Control.ElectricalSystem.TCMSAPSCBTripCmd
  In Bus Element54 : Inport  Port=6  PortName=TCMSSystemFB  Element=Control.ElectricalSystem.TCMSFDSCBTripCmd
  In Bus Element55 : Inport  Port=6  PortName=TCMSSystemFB  Element=Control.ElectricalSystem.TCMSHVAC1CBTripCmd
  In Bus Element56 : Inport  Port=6  PortName=TCMSSystemFB  Element=Control.ElectricalSystem.TCMSHVAC2CBTripCmd
  AND : Logic  AllPortsSameDT=off  OutDataTypeStr=boolean
  Bus Creator1 : BusCreator  Inputs=27  OutDataTypeStr=Bus: BD_SimIntegration_Faults_IOControls  NonVirtualBus=on
  Bus Selector : BusSelector  OutputSignals=PneumaticsFaults.ORDIntervention
  Bus Selector1 : BusSelector  OutputSignals=PressureSwitches.PS2
  ControlStateFault{,1..3} (4 alike) : IOStateMachinesLib/ControlStateFault  ControlType=Toggle  FltStVal=0  NormalStVal=1  ReturnToNormalState=on
      settings: SourceProductName=IO State Machines
  Data Type Conversion{,1..54} (55 alike) : DataTypeConversion
  IRQStateMachine{,1..21} (22 alike) : IOStateMachinesLib/IRQStateMachine  ControlType=Toggle  FltStVal=0  NormalStVal=1  ReturnToNormalState=on  TriggerContinously=off
      settings: SourceProductName=IO State Machines
  OR : Logic  Operator=OR  AllPortsSameDT=off  OutDataTypeStr=boolean
  Rate Transition{1..4} (4 alike) : RateTransition
  Subsystem : Subsystem
  Subsystem1 : Subsystem
  Subsystem2 : Subsystem
  Subsystem3 : Subsystem
  Subsystem4 : Subsystem
  Subsystem5 : Subsystem
  Subsystem6 : Subsystem
  Subsystem7 : Subsystem
  Subsystem8 : Subsystem
  Subsystem9 : Subsystem
  Terminator{,1..15,17..18,20..30} (29 alike) : Terminator
  Unit Delay1 : UnitDelay  SampleTime=-1  HasFrameUpgradeWarning=on
  Out1 : Outport
  wires:
  IRQStateMachine/2 -> Terminator/1
  In Bus Element5/1 -> Data Type Conversion/1
  In Bus Element6/1 -> IRQStateMachine/2
  Data Type Conversion/1 -> IRQStateMachine/1
  IRQStateMachine/1 -> Bus Creator1/1  "CCMCBInternalRequest"
  Bus Creator1/1 -> Out1/1
  IRQStateMachine1/1 -> Bus Creator1/2  "WWCBInternalRequest"
  Data Type Conversion1/1 -> IRQStateMachine1/1
  In Bus Element/1 -> IRQStateMachine1/2
  In Bus Element3/1 -> Data Type Conversion1/1
  IRQStateMachine1/2 -> Terminator1/1
  IRQStateMachine2/2 -> Terminator2/1
  In Bus Element2/1 -> Data Type Conversion2/1
  In Bus Element1/1 -> IRQStateMachine2/2
  Data Type Conversion2/1 -> IRQStateMachine2/1
  IRQStateMachine2/1 -> Bus Creator1/3  "CELCBInternalRequest"
  In Bus Element8/1 -> Data Type Conversion3/1
  Data Type Conversion3/1 -> IRQStateMachine3/1
  OR/1 -> Data Type Conversion6/1
  In Bus Element4/1 -> Data Type Conversion4/1
  In Bus Element7/1 -> Data Type Conversion5/1
  IRQStateMachine3/2 -> Terminator3/1
  IRQStateMachine3/1 -> Bus Creator1/4  "HLCBInternalRequest"
  Data Type Conversion4/1 -> OR/1
  Data Type Conversion5/1 -> OR/2
  Data Type Conversion6/1 -> IRQStateMachine3/2
  In Bus Element27/1 -> Data Type Conversion7/1
  IRQStateMachine4/2 -> Terminator4/1
  IRQStateMachine4/1 -> Bus Creator1/5  "MCBPAGroupOpenInternalRequest"
  In Bus Element18/1 -> Terminator13/1
  In Bus Element19/1 -> Terminator14/1
  In Bus Element20/1 -> Terminator15/1
  Data Type Conversion7/1 -> IRQStateMachine4/1
  Data Type Conversion8/1 -> IRQStateMachine4/2
  Subsystem/1(Out1) -> Data Type Conversion8/1
  In Bus Element32/1 -> Subsystem/1(InputControlStates)
  In Bus Element29/1 -> Subsystem1/1(InputControlStates)
  Subsystem1/1(Out1) -> Data Type Conversion10/1
  Data Type Conversion10/1 -> IRQStateMachine5/2
  Data Type Conversion9/1 -> IRQStateMachine5/1
  IRQStateMachine5/1 -> Bus Creator1/6  "MCB110VDCGroupOpenInternalRequest"
  IRQStateMachine5/2 -> Terminator23/1
  In Bus Element15/1 -> Data Type Conversion9/1
  In Bus Element30/1 -> Data Type Conversion12/1
  IRQStateMachine6/2 -> Terminator24/1
  IRQStateMachine6/1 -> Bus Creator1/7  "MCBLightGroupOpenInternalRequest"
  Data Type Conversion12/1 -> IRQStateMachine6/1
  Data Type Conversion11/1 -> IRQStateMachine6/2
  Subsystem2/1(Out1) -> Data Type Conversion11/1
  In Bus Element31/1 -> Subsystem2/1(InputControlStates)
  In Bus Element34/1 -> Subsystem3/1(InputControlStates)
  Subsystem3/1(Out1) -> Data Type Conversion13/1
  Data Type Conversion13/1 -> IRQStateMachine7/2
  Data Type Conversion14/1 -> IRQStateMachine7/1
  IRQStateMachine7/1 -> Bus Creator1/8  "MCBLightSaloonGroupOpenInternalRequest"
  IRQStateMachine7/2 -> Terminator25/1
  In Bus Element28/1 -> Data Type Conversion14/1
  In Bus Element22/1 -> Data Type Conversion16/1
  IRQStateMachine8/2 -> Terminator26/1
  IRQStateMachine8/1 -> Bus Creator1/9  "MCBDoorGroupOpenInternalRequest"
  Data Type Conversion16/1 -> IRQStateMachine8/1
  Data Type Conversion15/1 -> IRQStateMachine8/2
  Subsystem4/1(Out1) -> Data Type Conversion15/1
  In Bus Element36/1 -> Subsystem4/1(InputControlStates)
  In Bus Element38/1 -> Subsystem5/1(InputControlStates)
  Subsystem5/1(Out1) -> Data Type Conversion17/1
  Data Type Conversion17/1 -> IRQStateMachine9/2
  Data Type Conversion18/1 -> IRQStateMachine9/1
  IRQStateMachine9/1 -> Bus Creator1/10  "MCBBrakeGroupOpenInternalRequest"
  IRQStateMachine9/2 -> Terminator27/1
  In Bus Element25/1 -> Data Type Conversion18/1
  In Bus Element33/1 -> Data Type Conversion20/1
  IRQStateMachine10/2 -> Terminator28/1
  IRQStateMachine10/1 -> Bus Creator1/11  "MCBAPSGroupOpenInternalRequest"
  Data Type Conversion20/1 -> IRQStateMachine10/1
  Data Type Conversion19/1 -> IRQStateMachine10/2
  Subsystem6/1(Out1) -> Data Type Conversion19/1
  In Bus Element40/1 -> Subsystem6/1(InputControlStates)
  In Bus Element42/1 -> Subsystem7/1(InputControlStates)
  Subsystem7/1(Out1) -> Data Type Conversion21/1
  Data Type Conversion21/1 -> IRQStateMachine11/2
  Data Type Conversion22/1 -> IRQStateMachine11/1
  IRQStateMachine11/1 -> Bus Creator1/12  "MCBTCMSGroupOpenInternalRequest"
  IRQStateMachine11/2 -> Terminator29/1
  In Bus Element26/1 -> Data Type Conversion22/1
  In Bus Element21/1 -> Data Type Conversion24/1
  IRQStateMachine12/2 -> Terminator30/1
  IRQStateMachine12/1 -> Bus Creator1/13  "MCBSignallingGroupOpenInternalRequest"
  Data Type Conversion24/1 -> IRQStateMachine12/1
  Data Type Conversion23/1 -> IRQStateMachine12/2
  Subsystem8/1(Out1) -> Data Type Conversion23/1
  In Bus Element44/1 -> Subsystem8/1(InputControlStates)
  In Bus Element16/1 -> Data Type Conversion25/1
  Data Type Conversion25/1 -> IRQStateMachine13/2
  Data Type Conversion26/1 -> IRQStateMachine13/1
  IRQStateMachine13/1 -> Bus Creator1/14  "CECBOpenInternalRequest"
  IRQStateMachine13/2 -> Terminator11/1
  In Bus Element10/1 -> Data Type Conversion26/1
  In Bus Element11/1 -> Data Type Conversion28/1
  IRQStateMachine14/2 -> Terminator12/1
  IRQStateMachine14/1 -> Bus Creator1/15  "ELCB1OpenInternalRequest"
  Data Type Conversion28/1 -> IRQStateMachine14/1
  Data Type Conversion27/1 -> IRQStateMachine14/2
  In Bus Element23/1 -> Data Type Conversion27/1
  In Bus Element35/1 -> Data Type Conversion29/1
  Data Type Conversion29/1 -> IRQStateMachine15/2
  Data Type Conversion30/1 -> IRQStateMachine15/1
  IRQStateMachine15/1 -> Bus Creator1/16  "ELCB2OpenInternalRequest"
  IRQStateMachine15/2 -> Terminator17/1
  In Bus Element12/1 -> Data Type Conversion30/1
  In Bus Element13/1 -> Data Type Conversion32/1
  IRQStateMachine16/2 -> Terminator18/1
  IRQStateMachine16/1 -> Bus Creator1/17  "ILCB1OpenInternalRequest"
  Data Type Conversion32/1 -> IRQStateMachine16/1
  Data Type Conversion31/1 -> IRQStateMachine16/2
  In Bus Element39/1 -> Data Type Conversion31/1
  In Bus Element43/1 -> Data Type Conversion33/1
  Data Type Conversion33/1 -> IRQStateMachine17/2
  Data Type Conversion34/1 -> IRQStateMachine17/1
  IRQStateMachine17/1 -> Bus Creator1/18  "ILCB2OpenInternalRequest"
  IRQStateMachine17/2 -> Terminator20/1
  In Bus Element14/1 -> Data Type Conversion34/1
  In Bus Element24/1 -> Data Type Conversion36/1
  IRQStateMachine18/2 -> Terminator21/1
  IRQStateMachine18/1 -> Bus Creator1/19  "APSCBOpenInternalRequest"
  Data Type Conversion36/1 -> IRQStateMachine18/1
  Data Type Conversion35/1 -> IRQStateMachine18/2
  In Bus Element37/1 -> Data Type Conversion35/1
  In Bus Element41/1 -> Data Type Conversion37/1
  Data Type Conversion37/1 -> IRQStateMachine19/2
  Data Type Conversion38/1 -> IRQStateMachine19/1
  IRQStateMachine19/1 -> Bus Creator1/20  "UCCBOpenInternalRequest"
  IRQStateMachine19/2 -> Terminator22/1
  In Bus Element9/1 -> Data Type Conversion38/1
  In Bus Element47/1 -> Data Type Conversion40/1
  IRQStateMachine20/2 -> Terminator5/1
  IRQStateMachine20/1 -> Bus Creator1/21  "PANCBOpenInternalRequest"
  Data Type Conversion40/1 -> IRQStateMachine20/1
  Data Type Conversion39/1 -> IRQStateMachine20/2
  In Bus Element45/1 -> Data Type Conversion39/1
  In Bus Element48/1 -> Subsystem9/1(InputControlStates)
  Subsystem9/1(Out1) -> Data Type Conversion41/1
  Data Type Conversion41/1 -> IRQStateMachine21/2
  Data Type Conversion42/1 -> IRQStateMachine21/1
  IRQStateMachine21/2 -> Terminator7/1
  In Bus Element17/1 -> Data Type Conversion42/1
  IRQStateMachine21/1 -> Bus Creator1/22  "MCBHVACGroupOpenInternalRequest"
  Unit Delay1/1 -> Data Type Conversion43/1
  FaultsIn/1 -> Bus Selector/1
  Bus Selector/1 -> AND/1  "<ORDIntervention>"
  Data Type Conversion43/1 -> Bus Creator1/23  "ORDPlungerInternalRequest"
  AND/1 -> Unit Delay1/1
  Bus Selector1/1 -> AND/2  "<PS2>"
  PneumaticSystemFB/1 -> Bus Selector1/1
  In Bus Element51/1 -> Data Type Conversion49/1
  In Bus Element49/1 -> Data Type Conversion47/1
  ControlStateFault/2 -> Terminator6/1
  ControlStateFault1/2 -> Terminator8/1
  ControlStateFault2/2 -> Terminator9/1
  ControlStateFault3/2 -> Terminator10/1
  ControlStateFault/1 -> Data Type Conversion54/1  "APSICBInternalRequest"
  Rate Transition2/1 -> Bus Creator1/25  "FDSCBInternalRequest"
  Rate Transition3/1 -> Bus Creator1/26  "SAC1CBInternalRequest"
  Rate Transition4/1 -> Bus Creator1/27  "SAC2CBInternalRequest"
  In Bus Element54/1 -> Data Type Conversion46/1
  In Bus Element55/1 -> Data Type Conversion48/1
  Data Type Conversion44/1 -> ControlStateFault/1
  Data Type Conversion45/1 -> ControlStateFault/2
  Data Type Conversion46/1 -> ControlStateFault1/1
  Data Type Conversion47/1 -> ControlStateFault1/2
  Data Type Conversion48/1 -> ControlStateFault2/1
  Data Type Conversion49/1 -> ControlStateFault2/2
  In Bus Element56/1 -> Data Type Conversion51/1
  In Bus Element50/1 -> ControlStateFault3/2
  In Bus Element53/1 -> Data Type Conversion44/1
  In Bus Element46/1 -> Data Type Conversion45/1
  Rate Transition1/1 -> Bus Creator1/24  "APSICBInternalRequest"
  ControlStateFault1/1 -> Data Type Conversion53/1  "FDSCBInternalRequest"
  ControlStateFault2/1 -> Data Type Conversion52/1  "SAC1CBInternalRequest"
  ControlStateFault3/1 -> Data Type Conversion50/1  "SAC2CBInternalRequest"
  Data Type Conversion50/1 -> Rate Transition4/1
  Data Type Conversion51/1 -> ControlStateFault3/1
  Data Type Conversion52/1 -> Rate Transition3/1
  Data Type Conversion53/1 -> Rate Transition2/1
  Data Type Conversion54/1 -> Rate Transition1/1

== system BEML_EMU/InputsInterface/FaultHandler/Subsystem/TCMSFaults ==
  In Bus Element1 : Inport  PortName=VehicleFaults  Element=MasterControllerandTrainLineIncongruence
  In Bus Element8 : Inport  PortName=VehicleFaults  Element=CommunicationErrorRIO1RIO2
  In Bus Element9 : Inport  PortName=VehicleFaults  Element=RIOMastershipError
  In Bus Element11 : Inport  PortName=VehicleFaults  Element=ER1MajorFault
  In Bus Element6 : Inport  PortName=VehicleFaults  Element=UnexpectedDoorOpeningDetectedByCC
  In Bus Element12 : Inport  PortName=VehicleFaults  Element=BECUPWRAndBRKCmdAtSameTime
  In Bus Element13 : Inport  PortName=VehicleFaults  Element=BECU2MinorFault
  In Bus Element14 : Inport  PortName=VehicleFaults  Element=BECUMajorFault
  In Bus Element15 : Inport  PortName=VehicleFaults  Element=BECUMajorFaultWired
  In Bus Element3 : Inport  Port=2  PortName=TrainFaults  Element=NeutralZoneVCBBackupFunctionActivated
  In Bus Element2 : Inport  Port=2  PortName=TrainFaults  Element=TCMSFailure
  In Bus Element4 : Inport  Port=2  PortName=TrainFaults  Element=TCMSDisplayHanged
  In Bus Element5 : Inport  Port=2  PortName=TrainFaults  Element=CCUCommunicationError
  In Bus Element : Inport  Port=2  PortName=TrainFaults  Element=TractionCutModeSelectorInATPATOUTO
  In Bus Element7 : Inport  Port=2  PortName=TrainFaults  Element=HighTractiveEffortRequired
  In Bus Element10 : Inport  Port=2  PortName=TrainFaults  Element=DynamicBrakeCutOut
  Bus Assignment : BusAssignment  AssignedSignals=MasterControllerandTrainLineIncongruence,TCMSDisplayHanged,TCMSFailure,NeutralZoneVCBBackupFunctionActivated,CCUCommunicationError,UnexpectedDoorOpeningDetectedByCC,RIO1Fault,RIO1RIO2Fault,ERFault,TractionCutModeSelectorInATPATOUTO,HighTractiveEffortRequired,DynamicBrakeCutOut,BECUPWRAndBRKCmdAtSameTime,BECU2MinorFault,BECUMajorFault,BECUMajorFaultWired
  Constant1 : Constant  Value=0  OutDataTypeStr=Bus: BD_TCMSSystem_In_Vehicle_Faults
  Data Type Conversion{1..6} (6 alike) : DataTypeConversion
  Out1 : Outport
  wires:
  In Bus Element1/1 -> Data Type Conversion1/1
  Bus Assignment/1 -> Out1/1
  Constant1/1 -> Bus Assignment/1
  Data Type Conversion1/1 -> Bus Assignment/2
  In Bus Element2/1 -> Data Type Conversion2/1
  Data Type Conversion2/1 -> Bus Assignment/4
  Data Type Conversion3/1 -> Bus Assignment/5
  In Bus Element3/1 -> Data Type Conversion3/1
  In Bus Element4/1 -> Data Type Conversion4/1
  Data Type Conversion4/1 -> Bus Assignment/3
  In Bus Element5/1 -> Data Type Conversion5/1
  Data Type Conversion5/1 -> Bus Assignment/6
  In Bus Element6/1 -> Data Type Conversion6/1
  Data Type Conversion6/1 -> Bus Assignment/7
  In Bus Element9/1 -> Bus Assignment/8
  In Bus Element8/1 -> Bus Assignment/9
  In Bus Element11/1 -> Bus Assignment/10
  In Bus Element/1 -> Bus Assignment/11
  In Bus Element7/1 -> Bus Assignment/12
  In Bus Element10/1 -> Bus Assignment/13
  In Bus Element12/1 -> Bus Assignment/14
  In Bus Element13/1 -> Bus Assignment/15
  In Bus Element14/1 -> Bus Assignment/16
  In Bus Element15/1 -> Bus Assignment/17

== system BEML_EMU/InputsInterface/FaultHandler/Subsystem/TractionFaults ==
  In Bus Element10 : Inport  PortName=VehicleFaults  Element=PCUFailure
  In Bus Element1 : Inport  PortName=VehicleFaults  Element=CIFailure
  In Bus Element2 : Inport  PortName=VehicleFaults  Element=CIIsolated
  In Bus Element3 : Inport  PortName=VehicleFaults  Element=CIMicroprocessorAbnormal
  In Bus Element4 : Inport  PortName=VehicleFaults  Element=CILocalCommunicationFailure
  In Bus Element5 : Inport  PortName=VehicleFaults  Element=CIGateSignalAbnormal
  In Bus Element6 : Inport  PortName=VehicleFaults  Element=CITCMSCommunicationFailure
  In Bus Element : Inport  PortName=VehicleFaults  Element=DCLinkOverVoltageLevel1
  In Bus Element7 : Inport  PortName=VehicleFaults  Element=DCLinkLowVoltageLevel1
  In Bus Element9 : Inport  PortName=VehicleFaults  Element=HeavyWheelSlip
  In Bus Element11 : Inport  PortName=VehicleFaults  Element=AKOpenFailure
  In Bus Element12 : Inport  PortName=VehicleFaults  Element=KOpenFailure
  In Bus Element16 : Inport  PortName=VehicleFaults  Element=DerailmentDetectedRightSide
  In Bus Element13 : Inport  PortName=VehicleFaults  Element=BogieDerailed
  In Bus Element14 : Inport  PortName=VehicleFaults  Element=WSPActiveBogie1
  In Bus Element15 : Inport  PortName=VehicleFaults  Element=BECU1FailureAllSpeedSensors
  In Bus Element8 : Inport  Port=2  PortName=TrainFaults  Element=DynamicBrakeCutOut
  Bus Assignment : BusAssignment  AssignedSignals=PCUFailure,CIFailure,CIIsolated,CIMicroprocessorAbnormal,CILocalCommunicationFailure,CIGateSignalAbnormal,CITCMSCommunicationFailure,DCLinkOverVoltageLevel1,DCLinkLowVoltageLevel1,HeavyWheelSlide,HeavyWheelSlip,CIAKOpenFailure,CIKOpenFailure,DerailmentDetectedRightSide,BogieDerailed,WSPActiveBogie1,BECU1FailureAllSpeedSensors
  Constant1 : Constant  Value=0  OutDataTypeStr=Bus: BD_TractionSystem_In_Faults
  Out1 : Outport
  wires:
  Constant1/1 -> Bus Assignment/1
  Bus Assignment/1 -> Out1/1
  In Bus Element10/1 -> Bus Assignment/2
  In Bus Element1/1 -> Bus Assignment/3
  In Bus Element2/1 -> Bus Assignment/4
  In Bus Element3/1 -> Bus Assignment/5
  In Bus Element4/1 -> Bus Assignment/6
  In Bus Element5/1 -> Bus Assignment/7
  In Bus Element6/1 -> Bus Assignment/8
  In Bus Element/1 -> Bus Assignment/9
  In Bus Element7/1 -> Bus Assignment/10
  In Bus Element8/1 -> Bus Assignment/11
  In Bus Element9/1 -> Bus Assignment/12
  In Bus Element11/1 -> Bus Assignment/13
  In Bus Element12/1 -> Bus Assignment/14
  In Bus Element16/1 -> Bus Assignment/15
  In Bus Element13/1 -> Bus Assignment/16
  In Bus Element14/1 -> Bus Assignment/17
  In Bus Element15/1 -> Bus Assignment/18
